simulink model "Observer"  (R2019a)
settings: Solver=VariableStepAuto  StartTime=0.0  StopTime=100  RelTol=1e-3
values from neighbouring files (symbols this model uses):
  A = [     -0.0447      5.6993       0         -9.8056     0       0.0004 ... (first row only)    [Altitude_AirSpeed.m]    (also in C.mat = [-0.0447 -0.0076 0.0293 0 0 0 5.6993 -1.4866 -12.1418 0 -50 ; N_uy_bar.mat = [-0.0447 -0.0076 0.0293 0 0 0 5.6993 -1.4866 -12.1418 0 -50 )
  B = [      0         1.7371 ... (first row only)    [Altitude_AirSpeed.m]    (also in C.mat = [0  1.7371; -0.3067  -0.0025; -40.6088  -0.2448; 0  0; 0  0;; N_uy_bar.mat = [0  1.7371; -0.3067  -0.0025; -40.6088  -0.2448; 0  0; 0  0;)
  C = [1 0 0 0 0 0 ... (first row only)    [Altitude_AirSpeed.m]    (also in C.mat = [1  0  0  0  0  0; 0  0  0  0  1  0]; N_uy_bar.mat = [1  0  0  0  0  0; 0  0  0  0  1  0])
  K = K_opt(:,1:6)    [Altitude_AirSpeed.m]
  Kf = K_opt(:,7:8)    [Altitude_AirSpeed.m]
  N_uy_bar = [N_bar(7, :); N_bar(8, :)]    [Altitude_AirSpeed.m]    (also in N_uy_bar.mat = [0.0023441981438  0; 0.00913644457561  0])
undefined symbols (not defined in the file or in its folder): A_observer, B_observer
settings Model: Creator=Santi  LastModifiedBy=rohit
settings DataIOCC: ReturnWorkspaceOutputs=off
settings DebuggingCC: ArithmeticOperatorsInVariantConditions=warning
settings SFSimCC: SimUseLocalCustomCode=off
settings RTWCC: RTWUseLocalCustomCode=off
settings CodeAppCC: StateflowObjectComments=on

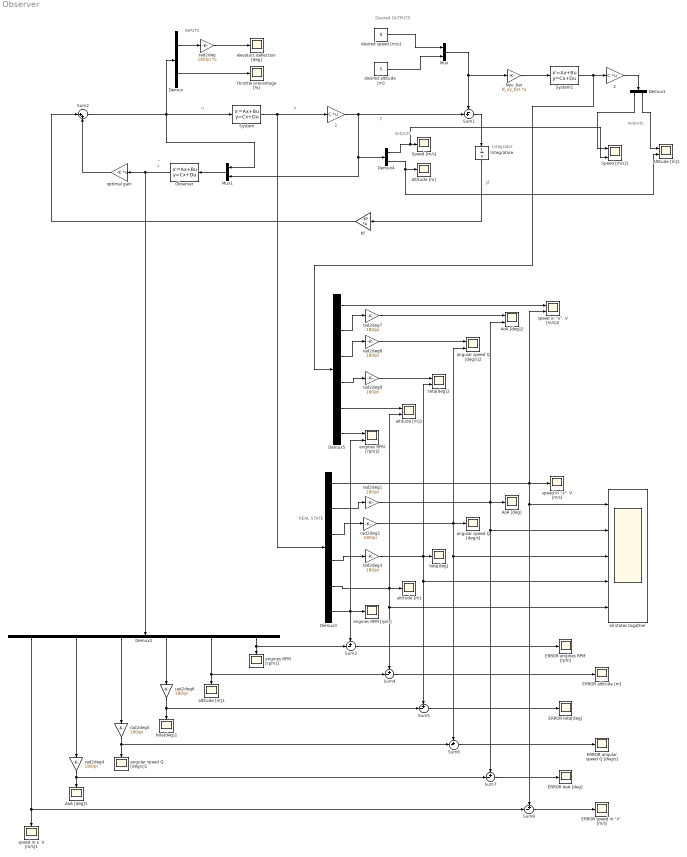
== system Observer ==
  note: ^
  note: x
  note: yf
  note: Integrator
  note: y
  note: x
  note: u
  note: outputs
  note: REAL STATE
  note: Desired OUTPUTS
  note: INPUTS
  note: outputs
  " 1" : Gain  Gain=C  Multiplication=Matrix(K*u)
  " 2" : Gain  Gain=C  Multiplication=Matrix(K*u)
  Altitude [m] : Scope
  Altitude [m]1 : Scope  NumInputPorts=2
  AoA [deg] : Scope
  AoA [deg]1 : Scope
  AoA [deg]2 : Scope  NumInputPorts=2
  Demux : Demux  Outputs=2
  Demux1 : Demux  Outputs=2
  Demux2 : Demux  Outputs=6
  Demux3 : Demux  Outputs=6
  Demux4 : Demux  Outputs=2
  Demux5 : Demux  Outputs=6
  ERROR AoA [deg] : Scope
  ERROR altitude [m] : Scope
  ERROR engines RPM [rpm] : Scope
  ERROR teta[deg] : Scope
  ERROR angular speed Q [deg/s] : Scope
  "ERROR speed in \"x\"  [m/s]" : Scope
  Integratore : Integrator
  Kf : Gain  Gain=-Kf  Multiplication=Matrix(K*u)
  Mux : Mux  Inputs=2
  Mux1 : Mux  Inputs=2
  Nyu_bar : Gain  Gain=N_uy_bar  Multiplication=Matrix(K*u)
  Observer : StateSpace  A=A_observer  B=B_observer  C=eye(6)  D=[zeros(6,4)]  InitialCondition=[0 0.05 0 0 0 0]
  Speed [m/s] : Scope
  Speed [m/s]1 : Scope  NumInputPorts=2
  Sum1 : Sum  Inputs=-+|
  Sum2 : Sum  Inputs=|++
  Sum{3..8} (6 alike) : Sum  Inputs=+-|
  System : StateSpace  A=A  B=B  C=eye(6)  D=[zeros(6,2)]  InitialCondition=[1 0 0 0 0 1]  ContinuousStateAttributes='system'
  System1 : StateSpace  A=A  B=B  C=eye(6)  D=[zeros(6,2)]  InitialCondition=[1 0 0 0 0 1]
  all states togather : Scope  NumInputPorts=5
  altitude [m] : Scope
  altitude [m]1 : Scope
  altitude [m]2 : Scope  NumInputPorts=2
  angular speed Q [deg/s] : Scope
  angular speed Q [deg/s]1 : Scope
  angular speed Q [deg/s]2 : Scope  NumInputPorts=2
  desired altitude  [m] : Constant  Value=5
  desired speed [m/s] : Constant  Value=0
  elevators deflection [deg] : Scope
  engines RPM [rpm] : Scope
  engines RPM [rpm]1 : Scope
  engines RPM [rpm]2 : Scope  NumInputPorts=2
  optimal gain : Gain  Gain=-K  Multiplication=Matrix(K*u)
  rad2deg : Gain  Gain=180/pi  Multiplication=Matrix(K*u)
  rad2deg{1..9} (9 alike) : Gain  Gain=180/pi
  speed in x  V [m/s]1 : Scope
  "speed in \"x\"  V [m/s]" : Scope
  "speed in \"x\"  V [m/s]2" : Scope  NumInputPorts=2
  teta[deg] : Scope
  teta[deg]1 : Scope
  teta[deg]2 : Scope  NumInputPorts=2
  throttle precentage [%] : Scope
  wires:
  System/1 -> " 1"/1, Demux3/1
  Sum1/1 -> Integratore/1
  " 1"/1 -> Mux1/2, Demux4/1, Sum1/2
  Integratore/1 -> Kf/1
  Kf/1 -> Sum2/1
  Demux3/6 -> engines RPM [rpm]2/2, engines RPM [rpm]/1, Sum3/1
  Demux3/5 -> altitude [m]2/2, altitude [m]/1, Sum4/1, all states togather/5
  rad2deg2/1 -> angular speed Q [deg/s]2/2, angular speed Q [deg/s]/1, Sum6/1, all states togather/3
  rad2deg1/1 -> AoA [deg]2/2, AoA [deg]/1, Sum7/1, all states togather/2
  Demux3/1 -> "speed in \"x\"  V [m/s]2"/2, "speed in \"x\"  V [m/s]"/1, Sum8/1, all states togather/1
  Demux3/2 -> rad2deg1/1
  Demux3/3 -> rad2deg2/1
  Demux3/4 -> rad2deg3/1
  desired speed [m/s]/1 -> Mux/1
  Mux/1 -> Nyu_bar/1, Sum1/1
  rad2deg/1 -> elevators deflection [deg]/1
  Demux/1 -> rad2deg/1
  Demux/2 -> throttle precentage [%]/1
  desired altitude  [m]/1 -> Mux/2
  Demux4/1 -> Speed [m/s]1/2, Speed [m/s]/1
  Nyu_bar/1 -> System1/1
  Demux1/2 -> Altitude [m]1/1
  Demux1/1 -> Speed [m/s]1/1
  " 2"/1 -> Demux1/1
  Demux4/2 -> Altitude [m]/1, Altitude [m]1/2
  Sum2/1 -> Mux1/1, Demux/1, System/1
  Mux1/1 -> Observer/1
  Observer/1 -> Demux2/1, optimal gain/1
  optimal gain/1 -> Sum2/2
  Demux2/6 -> Sum3/2, engines RPM [rpm]1/1
  Demux2/5 -> Sum4/2, altitude [m]1/1
  rad2deg6/1 -> Sum5/2, teta[deg]1/1
  rad2deg5/1 -> Sum6/2, angular speed Q [deg/s]1/1
  rad2deg4/1 -> AoA [deg]1/1, Sum7/2
  Demux2/1 -> Sum8/2, speed in x  V [m/s]1/1
  Demux2/2 -> rad2deg4/1
  Demux2/3 -> rad2deg5/1
  Demux2/4 -> rad2deg6/1
  Sum3/1 -> ERROR engines RPM [rpm]/1
  Sum4/1 -> ERROR altitude [m]/1
  Sum5/1 -> ERROR teta[deg]/1
  Sum6/1 -> ERROR angular speed Q [deg/s]/1
  Sum7/1 -> ERROR AoA [deg]/1
  Sum8/1 -> "ERROR speed in \"x\"  [m/s]"/1
  rad2deg3/1 -> teta[deg]2/2, teta[deg]/1, Sum5/1, all states togather/4
  System1/1 -> Demux5/1, " 2"/1
  Demux5/6 -> engines RPM [rpm]2/1
  Demux5/5 -> altitude [m]2/1
  rad2deg8/1 -> angular speed Q [deg/s]2/1
  rad2deg7/1 -> AoA [deg]2/1
  Demux5/1 -> "speed in \"x\"  V [m/s]2"/1
  Demux5/2 -> rad2deg7/1
  Demux5/3 -> rad2deg8/1
  Demux5/4 -> rad2deg9/1
  rad2deg9/1 -> teta[deg]2/1
